simulink model "untitled12013"  (R2013b)
settings: Solver=ode45  StartTime=0.0  StopTime=10.0  RelTol=1e-3
settings Model: Creator=darsan13  LastModifiedBy=darsan13

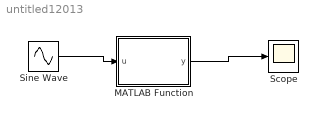
== system untitled12013 ==
  MATLAB Function : MATLAB Function  TreatAsAtomicUnit=on
  Scope : Scope
  Sine Wave : Sin  SampleTime=0
  wires:
  Sine Wave/1 -> MATLAB Function/1(u)
  MATLAB Function/1(y) -> Scope/1

== matlab function untitled12013/MATLAB Function ==
  data: u input; y output
function y = fcn(u)
%#codegen

y = 34*u;
